simulink model "untitled"  (R2024b)
settings: Solver=VariableStepAuto  StartTime=0.0  StopTime=10.0  RelTol=1e-3
values from neighbouring files (symbols this model uses):
  aalpha = Km / Ra    (= 0.4)    [untitleyd.m]
  f = 0.2    [untitleyd.m]
  J = 1    [untitleyd.m]
  Ka = 0.05    [untitleyd.m]
  Kb = 0.5    [untitleyd.m]
  Kt = 0    [untitleyd.m]
settings Model: Creator=aminh  LastModifiedBy=aminh

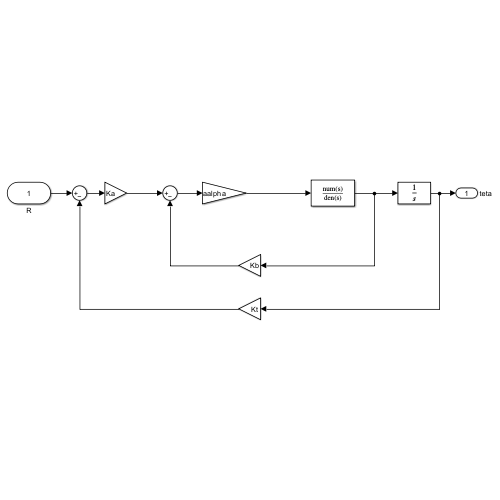
[thumbnail: Simulink's stored preview of the top-level diagram]
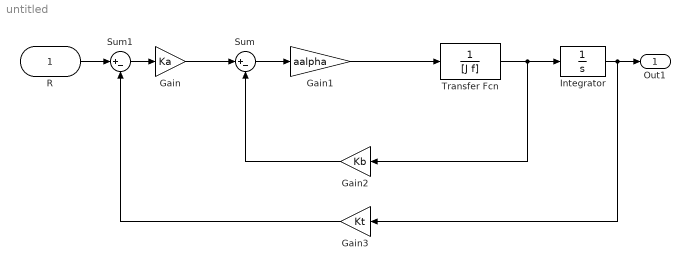
== system untitled ==
  R : Inport
  Gain : Gain  Gain=Ka
  Gain1 : Gain  Gain=aalpha
  Gain2 : Gain  Gain=Kb
  Gain3 : Gain  Gain=Kt
  Integrator : Integrator
  Sum : Sum  Inputs=|+-
  Sum1 : Sum  Inputs=|+-
  Transfer Fcn : TransferFcn  Denominator=[J f]
  Out1 : Outport  SignalName=teta
  wires:
  Gain/1 -> Sum/1
  Sum/1 -> Gain1/1
  Transfer Fcn/1 -> Gain2/1, Integrator/1
  Integrator/1 -> Gain3/1, Out1/1
  Gain2/1 -> Sum/2
  Gain1/1 -> Transfer Fcn/1
  Sum1/1 -> Gain/1
  R/1 -> Sum1/1
  Gain3/1 -> Sum1/2
